simulink model "SubsistemaSenalizacion"  (R2023b)
settings: Solver=VariableStepAuto  StartTime=0.0  StopTime=10.0  RelTol=1e-3
libraries: arduinolib x3, simulink x2
settings Model: Creator=manu_  LastModifiedBy=manu_

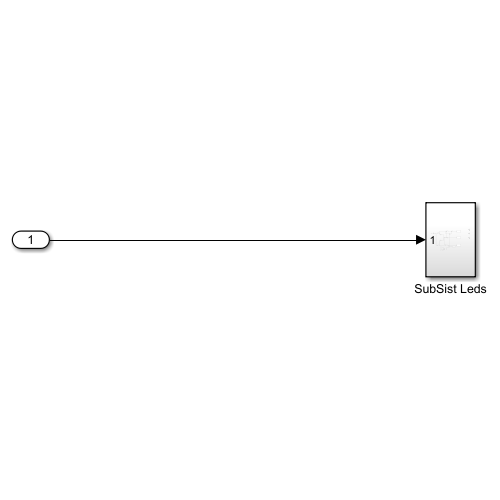
[thumbnail: Simulink's stored preview of the top-level diagram]
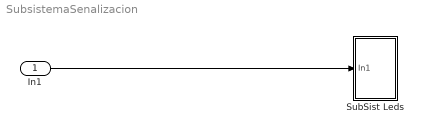
== system SubsistemaSenalizacion ==
  In1 : Inport
  SubSist Leds : Subsystem
  wires:
  In1/1 -> SubSist Leds/1(In1)

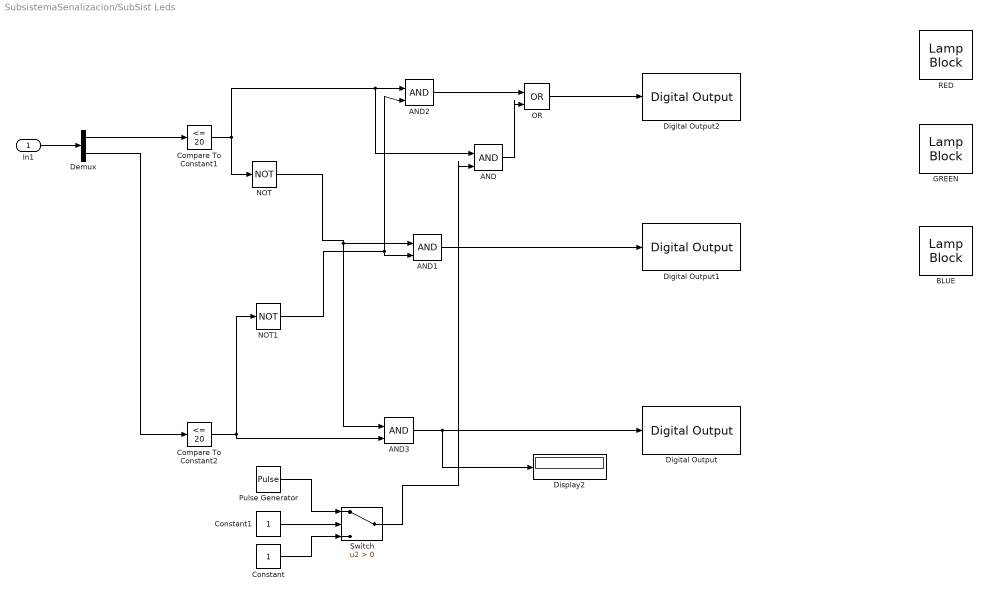
== system SubsistemaSenalizacion/SubSist Leds ==
  In1 : Inport
  AND{,1..3} (4 alike) : Logic  IconShape=distinctive  AllPortsSameDT=off  OutDataTypeStr=boolean
  BLUE : LampBlock  LabelPosition=Hide
  Compare To Constant1 : simulink/Logic and Bit Operations/Compare To Constant  relop=<=  const=20  OutDataTypeStr=boolean
  Compare To Constant2 : simulink/Logic and Bit Operations/Compare To Constant  relop=<=  const=20  OutDataTypeStr=boolean
  Constant : Constant
  Constant1 : Constant
  Demux : Demux  Outputs=2
  Digital Output : arduinolib/Digital Output  pinNumber=53  Direction=output  blockPlatform=arduino
  Digital Output1 : arduinolib/Digital Output  pinNumber=51  Direction=output  blockPlatform=arduino
  Digital Output2 : arduinolib/Digital Output  pinNumber=49  Direction=output  blockPlatform=arduino
  Display2 : Display
  GREEN : LampBlock  LabelPosition=Hide
  NOT : Logic  Operator=NOT  IconShape=distinctive  AllPortsSameDT=off  OutDataTypeStr=boolean
  NOT1 : Logic  Operator=NOT  IconShape=distinctive  AllPortsSameDT=off  OutDataTypeStr=boolean
  OR : Logic  Operator=OR  IconShape=distinctive  AllPortsSameDT=off  OutDataTypeStr=boolean
  Pulse Generator : DiscretePulseGenerator  PulseType=Time based  PulseWidth=50
  RED : LampBlock  LabelPosition=Hide
  Switch : Switch  Criteria=u2 > Threshold  SaturateOnIntegerOverflow=off  InputSameDT=off
  wires:
  OR/1 -> Digital Output2/1
  AND3/1 -> Display2/1, Digital Output/1
  AND2/1 -> OR/1
  Compare To Constant2/1 -> NOT1/1, AND3/2
  NOT1/1 -> AND2/2, AND1/2
  AND/1 -> OR/2
  Constant1/1 -> Switch/2
  Demux/1 -> Compare To Constant1/1
  NOT/1 -> AND3/1, AND1/1
  AND1/1 -> Digital Output1/1
  In1/1 -> Demux/1
  Compare To Constant1/1 -> AND/1, AND2/1, NOT/1
  Pulse Generator/1 -> Switch/1
  Constant/1 -> Switch/3
  Switch/1 -> AND/2
  Demux/2 -> Compare To Constant2/1
